simulink library "sFunctionLibrary"  (R2025b)
settings: Solver=VariableStepAuto  StartTime=0.0  StopTime=10.0  RelTol=1e-3
settings Model: Creator=AdamY  LastModifiedBy=palla

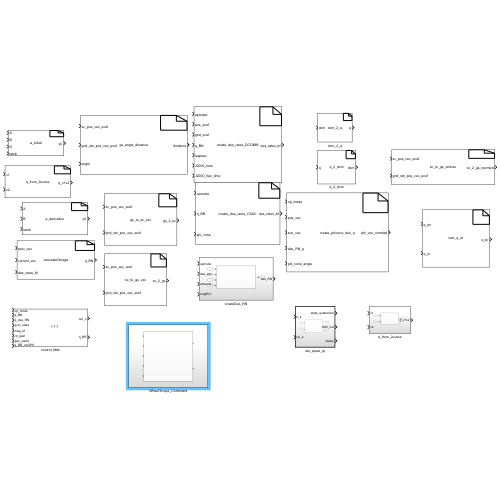
[thumbnail: Simulink's stored preview of the top-level diagram]
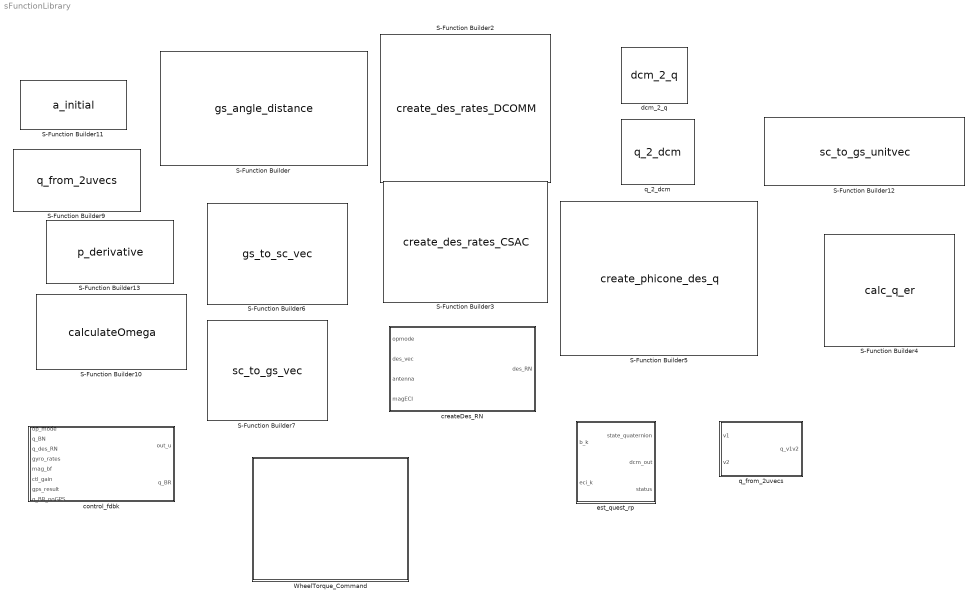
== system sFunctionLibrary ==
  S-Function Builder : S-Function  FunctionName=gs_angle_distance  SFunctionModules=gs_angle_distance_wrapper.c mtx conversions ref_rotation att_det global  SFunctionDeploymentMode=off  EnableBusSupport=off  mask(S-Function Builder){}
      mask help: Simulink:masks:SFunctionBuilder_MD
      mask init:
      | val = [[.9  0.75 0.75 1 1 .9 .9 1]',[1 1 0.75 0.75 .9 .9 1 .9]'];try , sys = get_param(gcb,'SfunBuilderFcnName');if isempty(sys), sys = get_param(gcb,'FunctionName'); end,catch, sys = get_param(gcb,'FunctionName'); end
      settings: CopyFcn=set_param(gcbh,'LinkStatus','none')  OpenFcn=sfunctionwizard(gcbh)
      mask Display:
      | plot(val(:,1),val(:,2))
      | disp(sys)
      | port_label('input',1,sprintf('%s', 'sc\_pos\_vec\_ecef'),'interpreter','tex')
      | port_label('input',2,sprintf('%s', 'gnd\_stn\_pos\_vec\_ecef'),'interpreter','tex')
      | port_label('input',3,sprintf('%s', 'angle'),'interpreter','tex')
      | port_label('output',1,sprintf('%s', 'distance'),'interpreter','tex')
  S-Function Builder10 : S-Function  FunctionName=calculateOmega  SFunctionModules=calculateOmega_wrapper.c mtx conversions ref_rotation att_det global  SFunctionDeploymentMode=off  EnableBusSupport=off  mask(S-Function Builder){}
      mask help: Simulink:masks:SFunctionBuilder_MD
      mask init: same as sFunctionLibrary/S-Function Builder
      settings: CopyFcn=set_param(gcbh,'LinkStatus','none')  OpenFcn=sfunctionwizard(gcbh)
      mask Display:
      | plot(val(:,1),val(:,2))
      | disp(sys)
      | port_label('input',1,sprintf('%s', 'prev\_vec'),'interpreter','tex')
      | port_label('input',2,sprintf('%s', 'current\_vec'),'interpreter','tex')
      | port_label('input',3,sprintf('%s', 'des\_rates\_bf'),'interpreter','tex')
      | port_label('output',1,sprintf('%s', 'q\_BN'),'interpreter','tex')
  S-Function Builder11 : S-Function  FunctionName=a_initial  SFunctionModules=a_initial_wrapper.c mtx conversions ref_rotation att_det global  SFunctionDeploymentMode=off  EnableBusSupport=off  mask(S-Function Builder){}
      mask help: Simulink:masks:SFunctionBuilder_MD
      mask init: same as sFunctionLibrary/S-Function Builder
      settings: CopyFcn=set_param(gcbh,'LinkStatus','none')  OpenFcn=sfunctionwizard(gcbh)
      mask Display:
      | plot(val(:,1),val(:,2))
      | disp(sys)
      | port_label('input',1,sprintf('%s', 'A'),'interpreter','tex')
      | port_label('input',2,sprintf('%s', 'B'),'interpreter','tex')
      | port_label('input',3,sprintf('%s', 'D'),'interpreter','tex')
      | port_label('input',4,sprintf('%s', 'lamb'),'interpreter','tex')
      | port_label('output',1,sprintf('%s', 'y0'),'interpreter','tex')
  S-Function Builder12 : S-Function  FunctionName=sc_to_gs_unitvec  SFunctionModules=sc_to_gs_unitvec_wrapper.c mtx conversions ref_rotation att_det global  SFunctionDeploymentMode=off  EnableBusSupport=off  mask(S-Function Builder){}
      mask help: Simulink:masks:SFunctionBuilder_MD
      mask init: same as sFunctionLibrary/S-Function Builder
      settings: CopyFcn=set_param(gcbh,'LinkStatus','none')  OpenFcn=sfunctionwizard(gcbh)
      mask Display:
      | plot(val(:,1),val(:,2))
      | disp(sys)
      | port_label('input',1,sprintf('%s', 'sc\_pos\_vec\_ecef'),'interpreter','tex')
      | port_label('input',2,sprintf('%s', 'gnd\_stn\_pos\_vec\_ecef'),'interpreter','tex')
      | port_label('output',1,sprintf('%s', 'sc\_2\_gs\_normlzd'),'interpreter','tex')
  S-Function Builder13 : S-Function  FunctionName=p_derivative  SFunctionModules=p_derivative_wrapper.c mtx conversions ref_rotation att_det global  SFunctionDeploymentMode=off  EnableBusSupport=off  mask(S-Function Builder){}
      mask help: Simulink:masks:SFunctionBuilder_MD
      mask init: same as sFunctionLibrary/S-Function Builder
      settings: CopyFcn=set_param(gcbh,'LinkStatus','none')  OpenFcn=sfunctionwizard(gcbh)
      mask Display:
      | plot(val(:,1),val(:,2))
      | disp(sys)
      | port_label('input',1,sprintf('%s', 'A'),'interpreter','tex')
      | port_label('input',2,sprintf('%s', 'B'),'interpreter','tex')
      | port_label('input',3,sprintf('%s', 'lamb'),'interpreter','tex')
      | port_label('output',1,sprintf('%s', 'y0'),'interpreter','tex')
  S-Function Builder2 : S-Function  FunctionName=create_des_rates_DCOMM  SFunctionModules=create_des_rates_DCOMM_wrapper.c mtx att_det global conversions ref_rotation  SFunctionDeploymentMode=off  EnableBusSupport=off  mask(S-Function Builder){}
      mask help: Simulink:masks:SFunctionBuilder_MD
      mask init: same as sFunctionLibrary/S-Function Builder
      settings: CopyFcn=set_param(gcbh,'LinkStatus','none')  OpenFcn=sfunctionwizard(gcbh)
      mask Display:
      | plot(val(:,1),val(:,2))
      | disp(sys)
      | port_label('input',1,sprintf('%s', 'opmode'),'interpreter','tex')
      | port_label('input',2,sprintf('%s', 'pos\_ecef'),'interpreter','tex')
      | port_label('input',3,sprintf('%s', 'gnd\_ecef'),'interpreter','tex')
      | port_label('input',4,sprintf('%s', 'q\_BN'),'interpreter','tex')
      | port_label('input',5,sprintf('%s', 'leapsec'),'interpreter','tex')
      | port_label('input',6,sprintf('%s', 'J2000\_time'),'interpreter','tex')
      | port_label('input',7,sprintf('%s', 'J2000\_frac\_time'),'interpreter','tex')
      | port_label('output',1,sprintf('%s', 'des\_rates\_bf'),'interpreter','tex')
  S-Function Builder3 : S-Function  FunctionName=create_des_rates_CSAC  SFunctionModules=create_des_rates_CSAC_wrapper.c mtx conversions ref_rotation att_det global  SFunctionDeploymentMode=off  EnableBusSupport=off  mask(S-Function Builder){}
      mask help: Simulink:masks:SFunctionBuilder_MD
      mask init: same as sFunctionLibrary/S-Function Builder
      settings: CopyFcn=set_param(gcbh,'LinkStatus','none')  OpenFcn=sfunctionwizard(gcbh)
      mask Display:
      | plot(val(:,1),val(:,2))
      | disp(sys)
      | port_label('input',1,sprintf('%s', 'opmode'),'interpreter','tex')
      | port_label('input',2,sprintf('%s', 'q\_BN'),'interpreter','tex')
      | port_label('input',3,sprintf('%s', 'phi\_cone'),'interpreter','tex')
      | port_label('output',1,sprintf('%s', 'des\_rates\_bf'),'interpreter','tex')
  S-Function Builder4 : S-Function  FunctionName=calc_q_er  SFunctionModules=calc_q_er_wrapper.c mtx conversions ref_rotation att_det global  SFunctionDeploymentMode=off  EnableBusSupport=off  mask(S-Function Builder){}
      mask help: Simulink:masks:SFunctionBuilder_MD
      mask init: same as sFunctionLibrary/S-Function Builder
      settings: CopyFcn=set_param(gcbh,'LinkStatus','none')  OpenFcn=sfunctionwizard(gcbh)
      mask Display:
      | plot(val(:,1),val(:,2))
      | disp(sys)
      | port_label('input',1,sprintf('%s', 'q\_bn'),'interpreter','tex')
      | port_label('input',2,sprintf('%s', 'q\_rn'),'interpreter','tex')
      | port_label('output',1,sprintf('%s', 'q\_br'),'interpreter','tex')
  S-Function Builder5 : S-Function  FunctionName=create_phicone_des_q  SFunctionModules=create_phicone_des_q_wrapper.c mtx conversions ref_rotation att_det global  SFunctionDeploymentMode=off  EnableBusSupport=off  mask(S-Function Builder){}
      mask help: Simulink:masks:SFunctionBuilder_MD
      mask init: same as sFunctionLibrary/S-Function Builder
      settings: CopyFcn=set_param(gcbh,'LinkStatus','none')  OpenFcn=sfunctionwizard(gcbh)
      mask Display:
      | plot(val(:,1),val(:,2))
      | disp(sys)
      | port_label('input',1,sprintf('%s', 'op\_mode'),'interpreter','tex')
      | port_label('input',2,sprintf('%s', 'pos\_vec'),'interpreter','tex')
      | port_label('input',3,sprintf('%s', 'sun\_vec'),'interpreter','tex')
      | port_label('input',4,sprintf('%s', 'des\_RN\_q'),'interpreter','tex')
      | port_label('input',5,sprintf('%s', 'phi\_cone\_angle'),'interpreter','tex')
      | port_label('output',1,sprintf('%s', 'phi\_vec\_normlzd'),'interpreter','tex')
  S-Function Builder6 : S-Function  FunctionName=gs_to_sc_vec  SFunctionModules=gs_to_sc_vec_wrapper.c mtx conversions ref_rotation att_det global  SFunctionDeploymentMode=off  EnableBusSupport=off  mask(S-Function Builder){}
      mask help: Simulink:masks:SFunctionBuilder_MD
      mask init: same as sFunctionLibrary/S-Function Builder
      settings: CopyFcn=set_param(gcbh,'LinkStatus','none')  OpenFcn=sfunctionwizard(gcbh)
      mask Display:
      | plot(val(:,1),val(:,2))
      | disp(sys)
      | port_label('input',1,sprintf('%s', 'sc\_pos\_vec\_ecef'),'interpreter','tex')
      | port_label('input',2,sprintf('%s', 'gnd\_stn\_pos\_vec\_ecef'),'interpreter','tex')
      | port_label('output',1,sprintf('%s', 'gs\_2\_sc'),'interpreter','tex')
  S-Function Builder7 : S-Function  FunctionName=sc_to_gs_vec  SFunctionModules=sc_to_gs_vec_wrapper.c mtx conversions ref_rotation att_det global  SFunctionDeploymentMode=off  EnableBusSupport=off  mask(S-Function Builder){}
      mask help: Simulink:masks:SFunctionBuilder_MD
      mask init: same as sFunctionLibrary/S-Function Builder
      settings: CopyFcn=set_param(gcbh,'LinkStatus','none')  OpenFcn=sfunctionwizard(gcbh)
      mask Display:
      | plot(val(:,1),val(:,2))
      | disp(sys)
      | port_label('input',1,sprintf('%s', 'sc\_pos\_vec\_ecef'),'interpreter','tex')
      | port_label('input',2,sprintf('%s', 'gnd\_stn\_pos\_vec\_ecef'),'interpreter','tex')
      | port_label('output',1,sprintf('%s', 'sc\_2\_gs'),'interpreter','tex')
  S-Function Builder9 : S-Function  FunctionName=q_from_2uvecs  SFunctionModules=q_from_2uvecs_wrapper.c mtx conversions ref_rotation att_det global  SFunctionDeploymentMode=off  EnableBusSupport=off  mask(S-Function Builder){}
      mask help: Simulink:masks:SFunctionBuilder_MD
      mask init: same as sFunctionLibrary/S-Function Builder
      settings: CopyFcn=set_param(gcbh,'LinkStatus','none')  OpenFcn=sfunctionwizard(gcbh)
      mask Display:
      | plot(val(:,1),val(:,2))
      | disp(sys)
      | port_label('input',1,sprintf('%s', 'v1'),'interpreter','tex')
      | port_label('input',2,sprintf('%s', 'v2'),'interpreter','tex')
      | port_label('output',1,sprintf('%s', 'q\_v1v2'),'interpreter','tex')
  WheelTorque_Command : Subsystem
  control_fdbk : Subsystem
      mask Display: image('ssc2023-01a.jpg');
  createDes_RN : Subsystem
  dcm_2_q : S-Function  FunctionName=dcm_2_q  SFunctionModules=dcm_2_q_wrapper.c mtx conversions ref_rotation att_det global  SFunctionDeploymentMode=off  EnableBusSupport=off  mask(S-Function Builder){}
      mask help: Simulink:masks:SFunctionBuilder_MD
      mask init: same as sFunctionLibrary/S-Function Builder
      settings: CopyFcn=set_param(gcbh,'LinkStatus','none')  OpenFcn=sfunctionwizard(gcbh)
      mask Display:
      | plot(val(:,1),val(:,2))
      | disp(sys)
      | port_label('input',1,sprintf('%s', 'dcm'),'interpreter','tex')
      | port_label('output',1,sprintf('%s', 'q'),'interpreter','tex')
  est_quest_rp : Subsystem  TreatAsAtomicUnit=on
  q_2_dcm : S-Function  FunctionName=q_2_dcm  SFunctionModules=q_2_dcm_wrapper.c mtx conversions ref_rotation att_det global  SFunctionDeploymentMode=off  EnableBusSupport=off  mask(S-Function Builder){}
      mask help: Simulink:masks:SFunctionBuilder_MD
      mask init: same as sFunctionLibrary/S-Function Builder
      settings: CopyFcn=set_param(gcbh,'LinkStatus','none')  OpenFcn=sfunctionwizard(gcbh)
      mask Display:
      | plot(val(:,1),val(:,2))
      | disp(sys)
      | port_label('input',1,sprintf('%s', 'q'),'interpreter','tex')
      | port_label('output',1,sprintf('%s', 'dcm'),'interpreter','tex')
  q_from_2uvecs : Subsystem

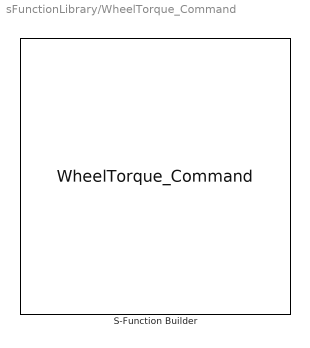
== system sFunctionLibrary/WheelTorque_Command ==
  S-Function Builder : S-Function  FunctionName=WheelTorque_Command  SFunctionModules=WheelTorque_Command_wrapper.c mtx rw_set global  SFunctionDeploymentMode=off  EnableBusSupport=off  mask(S-Function Builder){}
      mask help: Simulink:masks:SFunctionBuilder_MD
      mask init: same as sFunctionLibrary/S-Function Builder
      settings: CopyFcn=set_param(gcbh,'LinkStatus','none')  OpenFcn=sfunctionwizard(gcbh)
      mask Display:
      | plot(val(:,1),val(:,2))
      | disp(sys)
      | port_label('input',1,sprintf('%s', 'wheel\_speeds'),'interpreter','tex')
      | port_label('input',2,sprintf('%s', 'mag\_bf'),'interpreter','tex')
      | port_label('input',3,sprintf('%s', 'GsValues'),'interpreter','tex')
      | port_label('input',4,sprintf('%s', 'disabled\_wheel'),'interpreter','tex')
      | port_label('input',5,sprintf('%s', 'out\_u'),'interpreter','tex')
      | port_label('output',1,sprintf('%s', 'pwm\_dipole'),'interpreter','tex')
      | port_label('output',2,sprintf('%s', 'rw\_torque'),'interpreter','tex')

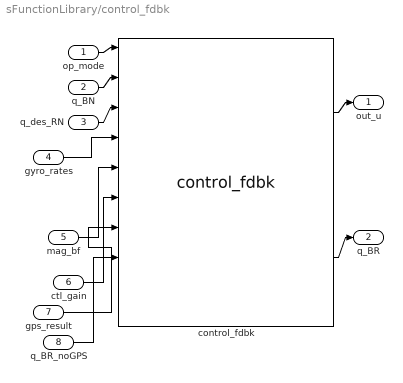
== system sFunctionLibrary/control_fdbk ==
  op_mode : Inport
  q_BN : Inport  Port=2
  q_des_RN : Inport  Port=3
  gyro_rates : Inport  Port=4
  mag_bf : Inport  Port=5
  ctl_gain : Inport  Port=6
  gps_result : Inport  Port=7
  q_BR_noGPS : Inport  Port=8
  control_fdbk : S-Function  FunctionName=control_fdbk  SFunctionModules=control_fdbk_wrapper.c mtx conversions ref_rotation global ctl_alg att_det  SFunctionDeploymentMode=off  EnableBusSupport=off  mask(S-Function Builder){}
      mask help: Simulink:masks:SFunctionBuilder_MD
      mask init: same as sFunctionLibrary/S-Function Builder
      settings: CopyFcn=set_param(gcbh,'LinkStatus','none')  OpenFcn=sfunctionwizard(gcbh)
      mask Display:
      | plot(val(:,1),val(:,2))
      | disp(sys)
      | port_label('input',1,sprintf('%s', 'op\_mode'),'interpreter','tex')
      | port_label('input',2,sprintf('%s', 'q\_BN'),'interpreter','tex')
      | port_label('input',3,sprintf('%s', 'q\_des\_RN'),'interpreter','tex')
      | port_label('input',4,sprintf('%s', 'gyro\_rates'),'interpreter','tex')
      | port_label('input',5,sprintf('%s', 'mag\_bf'),'interpreter','tex')
      | port_label('input',6,sprintf('%s', 'ctl\_gain'),'interpreter','tex')
      | port_label('input',7,sprintf('%s', 'gps\_result\_override'),'interpreter','tex')
      | port_label('input',8,sprintf('%s', 'q\_BR\_noGPS'),'interpreter','tex')
      | port_label('input',9,sprintf('%s', 'des\_rates'),'interpreter','tex')
      | port_label('input',10,sprintf('%s', 'u1'),'interpreter','tex')
      | port_label('output',1,sprintf('%s', 'out\_u'),'interpreter','tex')
      | port_label('output',2,sprintf('%s', 'q\_BR'),'interpreter','tex')
  out_u : Outport
  q_BR : Outport  Port=2
  wires:
  gyro_rates/1 -> control_fdbk/4
  op_mode/1 -> control_fdbk/1
  q_BN/1 -> control_fdbk/2
  mag_bf/1 -> control_fdbk/5
  ctl_gain/1 -> control_fdbk/6
  q_des_RN/1 -> control_fdbk/3
  control_fdbk/1 -> out_u/1
  control_fdbk/2 -> q_BR/1
  gps_result/1 -> control_fdbk/7
  q_BR_noGPS/1 -> control_fdbk/8

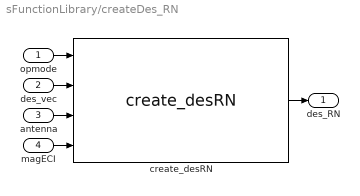
== system sFunctionLibrary/createDes_RN ==
  opmode : Inport
  des_vec : Inport  Port=2
  antenna : Inport  Port=3
  magECI : Inport  Port=4
  create_desRN : S-Function  FunctionName=create_desRN  SFunctionModules=create_desRN_wrapper.c mtx conversions ref_rotation att_det global  SFunctionDeploymentMode=off  EnableBusSupport=off  mask(S-Function Builder){}
      mask help: Simulink:masks:SFunctionBuilder_MD
      mask init: same as sFunctionLibrary/S-Function Builder
      settings: CopyFcn=set_param(gcbh,'LinkStatus','none')  OpenFcn=sfunctionwizard(gcbh)
      mask Display:
      | plot(val(:,1),val(:,2))
      | disp(sys)
      | port_label('input',1,sprintf('%s', 'opmode'),'interpreter','tex')
      | port_label('input',2,sprintf('%s', 'des\_vec'),'interpreter','tex')
      | port_label('input',3,sprintf('%s', 'antenna'),'interpreter','tex')
      | port_label('input',4,sprintf('%s', 'b\_eci'),'interpreter','tex')
      | port_label('output',1,sprintf('%s', 'des\_RN'),'interpreter','tex')
  des_RN : Outport
  wires:
  antenna/1 -> create_desRN/3
  create_desRN/1 -> des_RN/1
  opmode/1 -> create_desRN/1
  des_vec/1 -> create_desRN/2
  magECI/1 -> create_desRN/4

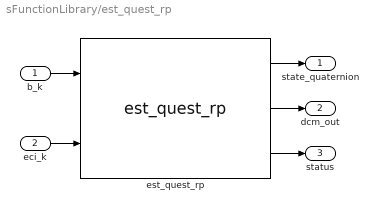
== system sFunctionLibrary/est_quest_rp ==
  b_k : Inport  OutDataTypeStr=single  PortDimensions=[3 2]
  eci_k : Inport  Port=2  OutDataTypeStr=single  PortDimensions=[3 2]
  est_quest_rp : S-Function  FunctionName=est_quest_rp  SFunctionModules=est_quest_rp_wrapper.c mtx att_det global conversions ref_rotation  SFunctionDeploymentMode=off  EnableBusSupport=off  mask(S-Function Builder){}
      mask help: Simulink:masks:SFunctionBuilder_MD
      mask init: same as sFunctionLibrary/S-Function Builder
      settings: CopyFcn=set_param(gcbh,'LinkStatus','none')  OpenFcn=sfunctionwizard(gcbh)
      mask Display:
      | plot(val(:,1),val(:,2))
      | disp(sys)
      | port_label('input',1,sprintf('%s', 'b\_k'),'interpreter','tex')
      | port_label('input',2,sprintf('%s', 'eci\_k'),'interpreter','tex')
      | port_label('output',1,sprintf('%s', 'state\_quaternion'),'interpreter','tex')
      | port_label('output',2,sprintf('%s', 'dcm\_out'),'interpreter','tex')
      | port_label('output',3,sprintf('%s', 'status'),'interpreter','tex')
  state_quaternion : Outport  OutDataTypeStr=single  PortDimensions=[4 1]
  dcm_out : Outport  Port=2  OutDataTypeStr=single  PortDimensions=[3 3]
  status : Outport  Port=3  OutDataTypeStr=int32  PortDimensions=1
  wires:
  b_k/1 -> est_quest_rp/1
  est_quest_rp/1 -> state_quaternion/1
  est_quest_rp/2 -> dcm_out/1
  est_quest_rp/3 -> status/1
  eci_k/1 -> est_quest_rp/2

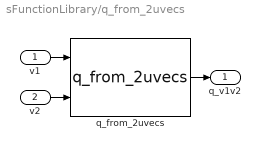
== system sFunctionLibrary/q_from_2uvecs ==
  v1 : Inport
  v2 : Inport  Port=2
  q_from_2uvecs : S-Function  FunctionName=q_from_2uvecs  SFunctionModules=q_from_2uvecs_wrapper.c att_det global conversions mtx ref_rotation  SFunctionDeploymentMode=off  EnableBusSupport=off  mask(S-Function Builder){}
      mask help: Simulink:masks:SFunctionBuilder_MD
      mask init: same as sFunctionLibrary/S-Function Builder
      settings: CopyFcn=set_param(gcbh,'LinkStatus','none')  OpenFcn=sfunctionwizard(gcbh)
      mask Display:
      | plot(val(:,1),val(:,2))
      | disp(sys)
      | port_label('input',1,sprintf('%s', 'v1'),'interpreter','tex')
      | port_label('input',2,sprintf('%s', 'v2'),'interpreter','tex')
      | port_label('output',1,sprintf('%s', 'q\_v1v2'),'interpreter','tex')
  q_v1v2 : Outport
  wires:
  v2/1 -> q_from_2uvecs/2
  v1/1 -> q_from_2uvecs/1
  q_from_2uvecs/1 -> q_v1v2/1
